simulink library "Mylibrary"  (Simulink 8.3)
settings: Solver=ode45  StartTime=0.0  StopTime=10.0  RelTol=1e-3
undefined symbols (not defined in the file or in its folder): Delay, epsilon, L, Mode, R, T_Trigger, tau_bar, Ts, Ts1, vd, Vehicle_Index, vp, x0, y0
undefined symbols (not defined in the file): d1, m1, psi20, Vx, Vy, x20, y20
libraries: Mylibrary x3
(part 1 of 3)
settings Model: Creator=hung  LastModifiedBy=hung  CovModelRefEnable=off  CovSFcnEnable=on

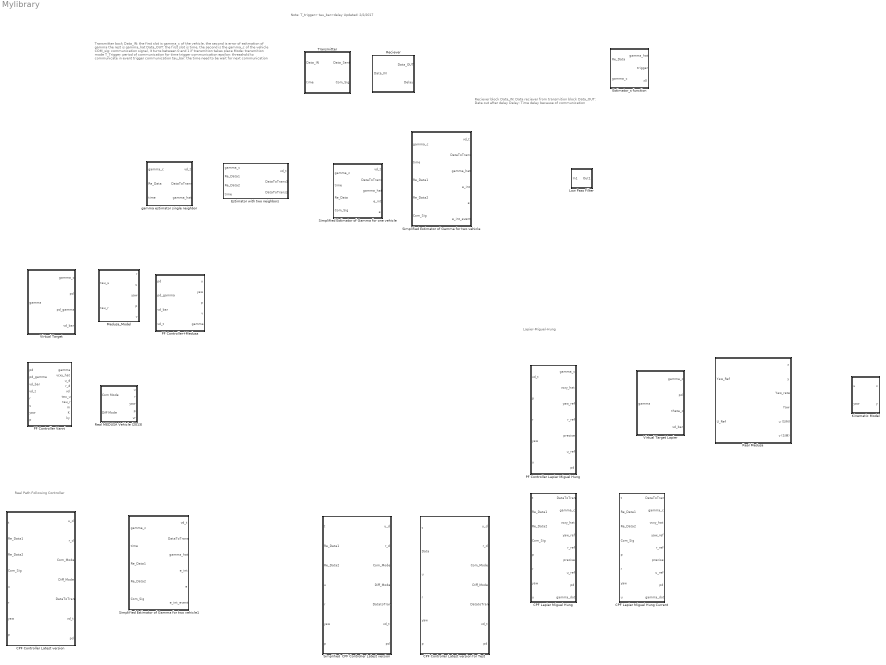
== system Mylibrary ==
  note: Lapier-Miguel-Hung
  note: Real Path Following Controller
  note: Note: T_trigger> tau_bar>delay
      | Updated: 2/2/2017
  note: Transmitter bock
      |
      | Data_IN: the first slot is gamma_c of the vehicle, the second is error of esitmation of gamma
      | the rest is gamma_hat
      | Data_OUT: the first slot is time, the second is the gamma_c of the vehicle
      | COM_sig: communication signal, it turns between 0 and 1 if transmition takes place
      |
      | Mode: transmition mode
      | T_Trigger: period of communication for time trigger communication
      | epsilon: threashold to communicate in event trigger communication
      | tau_bar: the time need to be wait for next communication
  note: Reciever block
      |
      | Data_IN: Data reciever from transmition block
      | Data_OUT: Data out after delay
      | Delay: Time delay because of communication
  " Real MEDUSA Vehicle (2013)" : Subsystem  mask{x0=0, y0=0, yaw0=0, u0=0, v0=0, r0=0, dist_u=0, dist_v=0, dist_r=0, Vcx=0, Vcy=0}
      mask prompts: dist_u "Disturbance in u"; dist_v "Disturbance in v"; dist_r "Disturbance in r"; Vcx "Current x"; Vcy "Current y"
  "CPF Controller Latest version  " : MATLAB Function  TreatAsAtomicUnit=on  mask{vp=0, L=0, m=0, d=0, R=0, tau_bar=0}
      settings: PermitHierarchicalResolution=ParametersOnly
  CPF Controller Latest version for Test : MATLAB Function  TreatAsAtomicUnit=on  mask{vp=0, L=0, m=0, d=0, R=0, tau_bar=0, Mode=0, T_Trigger=0, Parameter9=0, V_Id=0}
      mask prompts: Parameter9 "epsilon"
      settings: PermitHierarchicalResolution=ParametersOnly
  "CPF Lapier Miguel Hung " : MATLAB Function  TreatAsAtomicUnit=on  mask{L=L, R=R, d=d1, vp=vp, m=m1, tau_bar=tau_bar}
      settings: PermitHierarchicalResolution=ParametersOnly
  CPF Lapier Miguel Hung Current : MATLAB Function  TreatAsAtomicUnit=on  mask{L=L, R=R, d=d1, vp=vp, m=m1, tau_bar=tau_bar}
      settings: PermitHierarchicalResolution=ParametersOnly
  Estimator with two neighbors : Subsystem  mask{tau_bar=0, Parameter2=0}
      mask prompts: Parameter2 "Mode"
  Estimator_s function : Subsystem
  Kinematic Model : Subsystem
  Low Pass Filter : Subsystem
  Medusa_Model : Subsystem  mask{x0=x20, y0=y20, yaw0=psi20, u0=0, v0=0, r0=0, dist_u=0, dist_v=0, dist_r=0, Vcx=Vx, Vcy=Vy}
      mask prompts: dist_u "Disturbance in u"; dist_v "Disturbance in v"; dist_r "Disturbance in r"; Vcx "Current x"; Vcy "Current y"
  "PF Controller Lapier Miguel Hung " : MATLAB Function  TreatAsAtomicUnit=on  mask{L=L, R=R, d=d1, vd=vd, m=m1}
      settings: PermitHierarchicalResolution=ParametersOnly
  "PF Controller Vanni " : MATLAB Function  TreatAsAtomicUnit=on
      settings: PermitHierarchicalResolution=ParametersOnly
  PF Controller+Medusa : Subsystem
  Real Medusa : Subsystem
  Reciever : Subsystem  TreatAsAtomicUnit=on  mask{Delay=Delay}
      mask Display: image('Diagram2.png');
  "Simplified  CPF Controller Latest version " : MATLAB Function  TreatAsAtomicUnit=on  mask{vp=0, L=0, m=0, d=0, R=0, tau_bar=0, Mode=0, T_Trigger=0, Parameter9=0}
      mask prompts: Parameter9 "epsilon"
      settings: PermitHierarchicalResolution=ParametersOnly
  Simplified Estimator of Gamma for one vehicle : Subsystem  mask{Parameter1=0, Parameter2=0, Parameter3=0}
      mask prompts: Parameter1 "Mode"; Parameter2 "vd"; Parameter3 "tau_bar"
  Simplified Estimator of Gamma for two vehicle : Subsystem  mask{Parameter1=0, Parameter2=0, Parameter3=0}
      mask prompts: Parameter1 "Mode"; Parameter2 "vd"; Parameter3 "tau_bar"
  Simplified Estimator of Gamma for two vehicle1 : Subsystem  AncestorBlock=Mylibrary/Simplified Estimator of Gamma for two vehicle  mask{Parameter1=0, Parameter2=0, Parameter3=0}
      mask prompts: Parameter1 "Mode"; Parameter2 "vd"; Parameter3 "tau_bar"
  "Transmitter " : Subsystem  TreatAsAtomicUnit=on  mask{Mode=Mode, T_Trigger=T_Trigger, epsilon=epsilon, tau_bar=tau_bar}
      settings: MinAlgLoopOccurrences=on
      mask Display: image('transmit.png');
  Virtual Target : Subsystem  AncestorBlock=Mylibrary/Virtual Target  mask{L=0, R=0, d=0, vd=0, m=0}
      mask prompts: L "L (Length of the first segment)"; R "R (Radius for circumference)"; d "d (Offset from x axis)"; vd "vd (Speed profile)"
  Virtual Target Lapier : Subsystem  mask{L=0, R=0, d=0, vd=0, m=0}
      mask prompts: L "L (Length of the first segment)"; R "R (Radius for circumference)"; d "d (Offset from x axis)"; vd "vd (Speed profile)"
  gamma estimator single neighbor : Subsystem  TreatAsAtomicUnit=on  mask{Vehicle_Index=0, N_Vehicle_Index=0, tau_bar=0, Parameter4=0}
      mask prompts: Parameter4 "Mode"

== system Mylibrary/ Real MEDUSA Vehicle (2013) ==
  Com Mode : Inport
  Diff Mode : Inport  Port=2
  Medusa : Subsystem
  Mode : Constant  Value=4
  Mux : Mux  Inputs=2
  Saturation : Saturate  UpperLimit=100  LowerLimit=-100
  Saturation1 : Saturate  UpperLimit=100  LowerLimit=-100
  u : Outport
  r : Outport  Port=2
  yaw : Outport  Port=3
  p : Outport  Port=4
  vr : Outport  Port=5
  wires:
  Mode/1 -> Medusa/3(InnerLoops)
  Medusa/4(Yaw) -> yaw/1
  Medusa/3(Yaw_rate) -> r/1
  Medusa/6(v (SIM)) -> vr/1
  Medusa/5(u (SIM)) -> u/1
  Mux/1 -> p/1
  Medusa/1(x) -> Mux/1
  Medusa/2(y) -> Mux/2
  Diff Mode/1 -> Saturation1/1
  Com Mode/1 -> Saturation/1
  Saturation/1 -> Medusa/2(U_Ref)
  Saturation1/1 -> Medusa/1(Yaw_Ref)

== system Mylibrary/Estimator with two neighbors ==
  gamma_c : Inport
  Re_Data1 : Inport  Port=2
  Re_Data2 : Inport  Port=3
  time : Inport  Port=4
  Constant : Constant  Value=Mode
  Estimator i-j : Subsystem
  Estimator i-j1 : Mylibrary/Estimator with two neighbors/Estimator i-j
  MATLAB Function : MATLAB Function  TreatAsAtomicUnit=on
      settings: PermitHierarchicalResolution=ParametersOnly
  vd_t : Outport
  DataToTrans1 : Outport  Port=2
  DataToTrans2 : Outport  Port=3
  wires:
  time/1 -> Estimator i-j1/3, Estimator i-j/3("time ")
  gamma_c/1 -> Estimator i-j1/1, MATLAB Function/1(gamma_c), Estimator i-j/1(gamma_c)
  Estimator i-j1/2 -> MATLAB Function/3(gamma_hat2)
  Estimator i-j1/1 -> DataToTrans2/1
  Estimator i-j/1(DataToTrans) -> DataToTrans1/1
  Re_Data2/1 -> MATLAB Function/5(Re_Data2), Estimator i-j1/2
  Re_Data1/1 -> MATLAB Function/4(Re_Data1), Estimator i-j/2(Re_Data)
  Estimator i-j/2(gamma_hat) -> MATLAB Function/2(gamma_hat1)
  MATLAB Function/1(vd_t) -> vd_t/1
  Constant/1 -> MATLAB Function/6(Mode)

== system Mylibrary/Estimator_s function ==
  Re_Data : Inport
  gamma_c : Inport  Port=2
  Demux : Demux  Outputs=5
  Integrator : Integrator  ExternalReset=rising  InitialConditionSource=external
  Mux : Mux  Inputs=3
  Mux1 : Mux  Inputs=2
  Mux2 : Mux  Inputs=2
  S-Function : S-Function  FunctionName=estimator  Parameters=tau_bar  SFunctionDeploymentMode=off  EnableBusSupport=off
  gamma_hat : Outport
  trigger : Outport  Port=2
  x0 : Outport  Port=3
  wires:
  Mux1/1 -> x0/1, Integrator/3
  Mux/1 -> S-Function/1
  Demux/4 -> Mux1/1
  Demux/3 -> trigger/1, Integrator/2
  Mux2/1 -> Integrator/1
  S-Function/1 -> Demux/1
  Integrator/1 -> Mux/3, gamma_hat/1
  Demux/1 -> Mux2/1
  Demux/2 -> Mux2/2
  Demux/5 -> Mux1/2
  Re_Data/1 -> Mux/1
  gamma_c/1 -> Mux/2

== system Mylibrary/Kinematic Model ==
  u : Inport
  yaw : Inport  Port=2
  Integrator : Integrator  InitialCondition=x0
  Integrator1 : Integrator  InitialCondition=y0
  Kinematic Model : MATLAB Function  TreatAsAtomicUnit=on
      settings: PermitHierarchicalResolution=ParametersOnly
  x : Outport
  y : Outport  Port=2
  wires:
  yaw/1 -> Kinematic Model/2(yaw)
  u/1 -> Kinematic Model/1(u)
  Integrator1/1 -> y/1
  Kinematic Model/1(x_dot) -> Integrator/1
  Kinematic Model/2(y_dot) -> Integrator1/1
  Integrator/1 -> x/1

== system Mylibrary/Low Pass Filter ==
  In1 : Inport
  Demux : Demux  Outputs=2
  Mux : Mux  Inputs=2
  Transfer Fcn : TransferFcn  Denominator=[.2 1]
  Transfer Fcn1 : TransferFcn  Denominator=[.2 1]
  Out1 : Outport
  wires:
  Demux/2 -> Transfer Fcn1/1
  In1/1 -> Demux/1
  Demux/1 -> Transfer Fcn/1
  Transfer Fcn/1 -> Mux/1
  Mux/1 -> Out1/1
  Transfer Fcn1/1 -> Mux/2

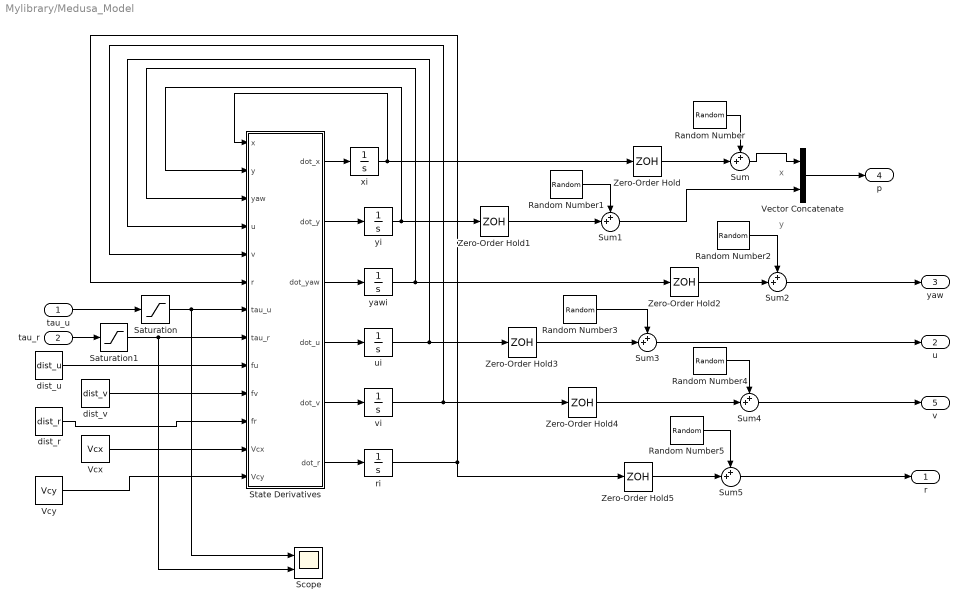
== system Mylibrary/Medusa_Model ==
  note: x
  note: y
  tau_u : Inport
  tau_r : Inport  Port=2
  Random Number : RandomNumber  Variance=.01  SampleTime=Ts1
  Random Number1 : RandomNumber  Variance=.01  SampleTime=Ts1
  Random Number2 : RandomNumber  Variance=.0001  SampleTime=Ts1
  Random Number3 : RandomNumber  Variance=.0001  SampleTime=Ts1
  Random Number4 : RandomNumber  SampleTime=Ts1
  Random Number5 : RandomNumber  Variance=0.0001  SampleTime=Ts1
  Saturation : Saturate  UpperLimit=100  LowerLimit=-100  ZeroCross=off
  Saturation1 : Saturate  UpperLimit=100  LowerLimit=-100  ZeroCross=off
  Scope : Scope  NumInputPorts=2
      settings: TimeRange=auto  MaxDataPoints=5000  SaveToWorkspace=off  SaveName=ScopeData3  YMin=-125.00000~-5  YMax=125.00000~5  SampleTime=-1
  State Derivatives : MATLAB Function  TreatAsAtomicUnit=on
      settings: PermitHierarchicalResolution=ParametersOnly
  Sum{,1..5} (6 alike) : Sum  Inputs=++|
  Vcx : Constant  Value=Vcx
  Vcy : Constant  Value=Vcy
  Vector Concatenate : Concatenate
  Zero-Order Hold{,1..5} (6 alike) : ZeroOrderHold  SampleTime=Ts1
  dist_r : Constant  Value=dist_r
  dist_u : Constant  Value=dist_u
  dist_v : Constant  Value=dist_v
  ri : Integrator  InitialCondition=r0
  ui : Integrator  InitialCondition=u0
  vi : Integrator  InitialCondition=v0
  xi : Integrator  InitialCondition=x0
  yawi : Integrator  InitialCondition=yaw0
  yi : Integrator  InitialCondition=y0
  r : Outport
  u : Outport  Port=2
  yaw : Outport  Port=3
  p : Outport  Port=4
  v : Outport  Port=5
  wires:
  State Derivatives/1(dot_x) -> xi/1
  State Derivatives/2(dot_y) -> yi/1
  State Derivatives/3(dot_yaw) -> yawi/1
  State Derivatives/4(dot_u) -> ui/1
  State Derivatives/5(dot_v) -> vi/1
  State Derivatives/6(dot_r) -> ri/1
  tau_u/1 -> Saturation/1
  tau_r/1 -> Saturation1/1
  dist_u/1 -> State Derivatives/9(fu)
  dist_v/1 -> State Derivatives/10(fv)
  dist_r/1 -> State Derivatives/11(fr)
  Vcx/1 -> State Derivatives/12(Vcx)
  Vcy/1 -> State Derivatives/13(Vcy)
  xi/1 -> Zero-Order Hold/1, State Derivatives/1(x)
  yi/1 -> Zero-Order Hold1/1, State Derivatives/2(y)
  ui/1 -> State Derivatives/4(u), Zero-Order Hold3/1
  vi/1 -> State Derivatives/5(v), Zero-Order Hold4/1
  ri/1 -> State Derivatives/6(r), Zero-Order Hold5/1
  Vector Concatenate/1 -> p/1
  Saturation/1 -> Scope/1, State Derivatives/7(tau_u)
  Saturation1/1 -> Scope/2, State Derivatives/8(tau_r)
  Sum1/1 -> Vector Concatenate/2
  Zero-Order Hold/1 -> Sum/2
  Sum/1 -> Vector Concatenate/1
  Random Number/1 -> Sum/1
  Zero-Order Hold1/1 -> Sum1/2
  Random Number1/1 -> Sum1/1
  yawi/1 -> Zero-Order Hold2/1, State Derivatives/3(yaw)
  Zero-Order Hold2/1 -> Sum2/2
  Sum2/1 -> yaw/1
  Random Number2/1 -> Sum2/1
  Zero-Order Hold3/1 -> Sum3/2
  Sum3/1 -> u/1
  Random Number3/1 -> Sum3/1
  Zero-Order Hold4/1 -> Sum4/2
  Sum4/1 -> v/1
  Random Number4/1 -> Sum4/1
  Zero-Order Hold5/1 -> Sum5/2
  Sum5/1 -> r/1
  Random Number5/1 -> Sum5/1

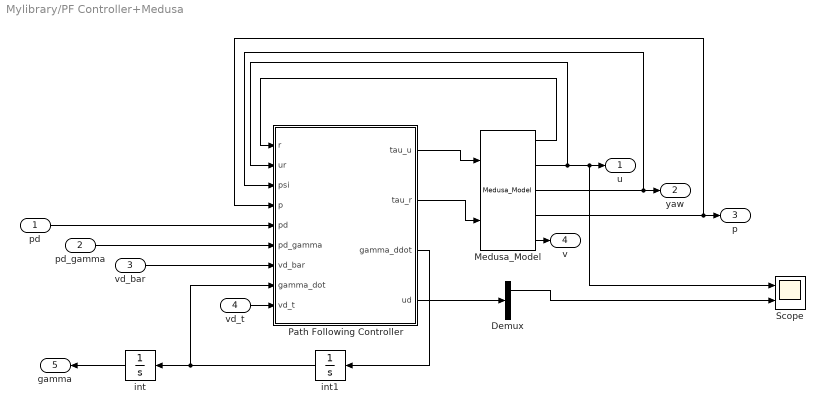
== system Mylibrary/PF Controller+Medusa ==
  pd : Inport
  pd_gamma : Inport  Port=2
  vd_bar : Inport  Port=3
  vd_t : Inport  Port=4
  Demux : Demux  Outputs=2
  Medusa_Model : Mylibrary/Medusa_Model  x0=x20  y0=y20  yaw0=psi20  u0=0  v0=0  r0=0  dist_u=0  dist_v=0  dist_r=0  Vcx=Vx  Vcy=Vy
  Path Following Controller : Subsystem
  Scope : Scope  NumInputPorts=2
      settings: TimeRange=auto  MaxDataPoints=5000  SaveToWorkspace=off  YMin=-1.16126~-5  YMax=10.45136~5  SampleTime=-1
  int : Integrator
  int1 : Integrator
  u : Outport
  yaw : Outport  Port=2
  p : Outport  Port=3
  v : Outport  Port=4
  gamma : Outport  Port=5
  wires:
  Medusa_Model/4 -> Path Following Controller/4(p), p/1
  Medusa_Model/3 -> Path Following Controller/3(psi), yaw/1
  Path Following Controller/3(gamma_ddot) -> int1/1
  pd/1 -> Path Following Controller/5(pd)
  int1/1 -> Path Following Controller/8(gamma_dot), int/1
  Path Following Controller/2(tau_r) -> Medusa_Model/2
  Medusa_Model/1 -> Path Following Controller/1(r)
  Medusa_Model/2 -> Path Following Controller/2(ur), Scope/1, u/1
  Path Following Controller/1(tau_u) -> Medusa_Model/1
  pd_gamma/1 -> Path Following Controller/6(pd_gamma)
  vd_bar/1 -> Path Following Controller/7(vd_bar)
  Medusa_Model/5 -> v/1
  vd_t/1 -> Path Following Controller/9(vd_t)
  int/1 -> gamma/1
  Path Following Controller/4(ud) -> Demux/1
  Demux/1 -> Scope/2

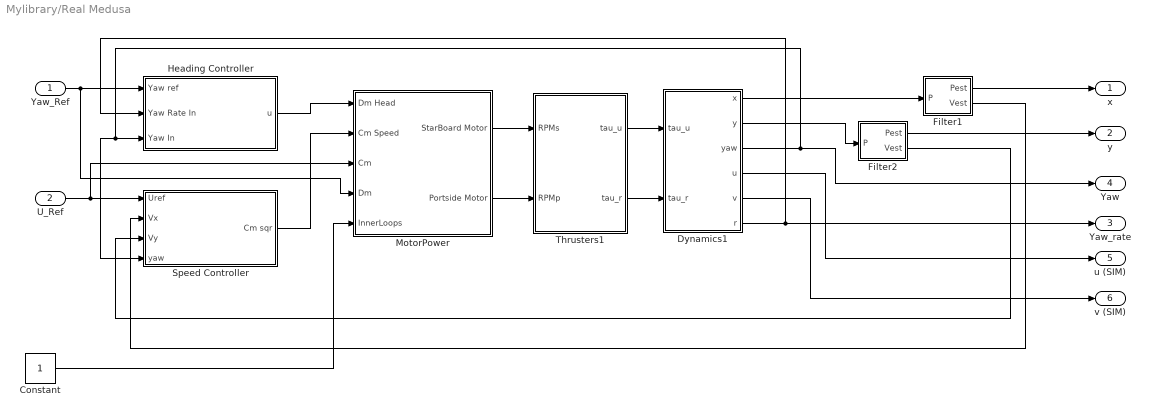
== system Mylibrary/Real Medusa ==
  Yaw_Ref : Inport
  U_Ref : Inport  Port=2
  Constant : Constant
  Dynamics1 : Subsystem  mask{x0=0, y0=0, yaw0=0, u0=0, v0=0, r0=0, dist_u=0, dist_v=0, dist_r=0, Vcx=0, Vcy=0}
      mask prompts: dist_u "Disturbance in u"; dist_v "Disturbance in v"; dist_r "Disturbance in r"; Vcx "Current x"; Vcy "Current y"
  Filter1 : Subsystem
  Filter2 : Subsystem
  Heading Controller : Subsystem  mask{Kp=45, Kd=110}
  MotorPower : Subsystem
  "Speed Controller " : Subsystem  mask{Kpu=60, Kiu=2, KSat=60}
      mask prompts: Kpu "Kp"; Kiu "Ki"; KSat "Common Mode Saturation"
  Thrusters1 : Subsystem
  x : Outport
  y : Outport  Port=2
  Yaw_rate : Outport  Port=3
  Yaw : Outport  Port=4
  u (SIM) : Outport  Port=5
  v (SIM) : Outport  Port=6
  wires:
  Thrusters1/1(tau_u) -> Dynamics1/1(tau_u)
  Thrusters1/2(tau_r) -> Dynamics1/2(tau_r)
  Dynamics1/1(x) -> Filter1/1(P)
  Dynamics1/2(y) -> Filter2/1(P)
  Dynamics1/3(yaw) -> Heading Controller/3(Yaw In), "Speed Controller "/4(yaw), Yaw/1
  MotorPower/1(StarBoard Motor) -> Thrusters1/1(RPMs)
  MotorPower/2(Portside Motor) -> Thrusters1/2(RPMp)
  Dynamics1/6(r) -> Heading Controller/2(Yaw Rate In), Yaw_rate/1
  Filter1/2(Vest) -> "Speed Controller "/2(Vx)
  Filter2/2(Vest) -> "Speed Controller "/3(Vy)
  "Speed Controller "/1(Cm sqr) -> MotorPower/2(Cm Speed)
  Yaw_Ref/1 -> Heading Controller/1(Yaw ref), MotorPower/4(Dm)
  Filter1/1(Pest) -> x/1
  Filter2/1(Pest) -> y/1
  U_Ref/1 -> "Speed Controller "/1(Uref), MotorPower/3(Cm)
  Heading Controller/1(u) -> MotorPower/1(Dm Head)
  Dynamics1/4(u) -> u (SIM)/1
  Dynamics1/5(v) -> v (SIM)/1
  Constant/1 -> MotorPower/5(InnerLoops)

== system Mylibrary/Reciever ==
  Data_IN : Inport  Priority=10
  Network Delay : MATLAB Function  Priority=11
      settings: PermitHierarchicalResolution=ParametersOnly
  Variable Time Delay1 : VariableTransportDelay  Priority=12  MaximumDelay=10  MaximumPoints=2048  ZeroDelay=on
  delay time : Constant  Value=Delay
  Data_OUT : Outport
  Delay : Outport  Port=2
  wires:
  Variable Time Delay1/1 -> Data_OUT/1
  delay time/1 -> Network Delay/2(DelayBound)
  Network Delay/1(delay_ins) -> Variable Time Delay1/2, Delay/1
  Data_IN/1 -> Variable Time Delay1/1, Network Delay/1(data)

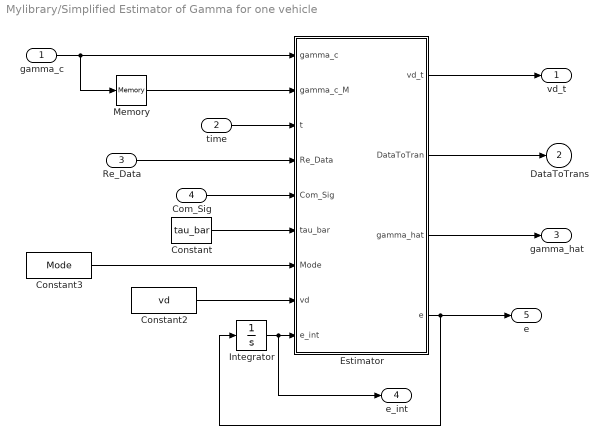
== system Mylibrary/Simplified Estimator of Gamma for one vehicle ==
  gamma_c : Inport
  "time " : Inport  Port=2
  Re_Data : Inport  Port=3
  Com_Sig : Inport  Port=4
  Constant : Constant  Value=tau_bar
  Constant2 : Constant  Value=vd
  Constant3 : Constant  Value=Mode
  Estimator : MATLAB Function  TreatAsAtomicUnit=on
      settings: PermitHierarchicalResolution=ParametersOnly
  Integrator : Integrator
  Memory : Memory
  vd_t : Outport
  DataToTrans : Outport  Port=2
  gamma_hat : Outport  Port=3
  e_int : Outport  Port=4
  e : Outport  Port=5
  wires:
  Constant3/1 -> Estimator/7(Mode)
  Estimator/2(DataToTran) -> DataToTrans/1
  Estimator/1(vd_t) -> vd_t/1
  Com_Sig/1 -> Estimator/5(Com_Sig)
  Re_Data/1 -> Estimator/4(Re_Data)
  "time "/1 -> Estimator/3(t)
  Constant/1 -> Estimator/6(tau_bar)
  Estimator/3(gamma_hat) -> gamma_hat/1
  Constant2/1 -> Estimator/8(vd)
  Estimator/4(e) -> e/1, Integrator/1
  Integrator/1 -> e_int/1, Estimator/9(e_int)
  gamma_c/1 -> Memory/1, Estimator/1(gamma_c)
  Memory/1 -> Estimator/2(gamma_c_M)

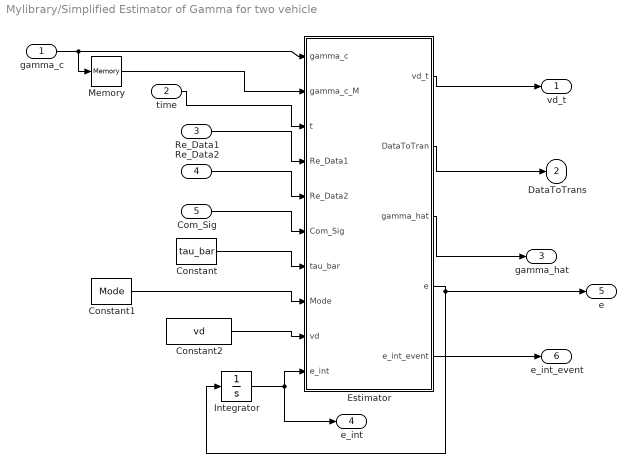
== system Mylibrary/Simplified Estimator of Gamma for two vehicle ==
  gamma_c : Inport
  "time " : Inport  Port=2
  Re_Data1 : Inport  Port=3
  Re_Data2 : Inport  Port=4
  Com_Sig : Inport  Port=5
  Constant : Constant  Value=tau_bar
  Constant1 : Constant  Value=Mode
  Constant2 : Constant  Value=vd
  Estimator : MATLAB Function  TreatAsAtomicUnit=on
      settings: PermitHierarchicalResolution=ParametersOnly
  Integrator : Integrator
  Memory : Memory
  vd_t : Outport
  DataToTrans : Outport  Port=2
  gamma_hat : Outport  Port=3
  e_int : Outport  Port=4
  e : Outport  Port=5
  e_int_event : Outport  Port=6
  wires:
  Estimator/1(vd_t) -> vd_t/1
  Estimator/3(gamma_hat) -> gamma_hat/1
  Constant2/1 -> Estimator/9(vd)
  Re_Data1/1 -> Estimator/4(Re_Data1)
  "time "/1 -> Estimator/3(t)
  Constant/1 -> Estimator/7(tau_bar)
  Com_Sig/1 -> Estimator/6(Com_Sig)
  Estimator/2(DataToTran) -> DataToTrans/1
  Re_Data2/1 -> Estimator/5(Re_Data2)
  Estimator/4(e) -> e/1, Integrator/1
  Integrator/1 -> e_int/1, Estimator/10(e_int)
  gamma_c/1 -> Memory/1, Estimator/1(gamma_c)
  Constant1/1 -> Estimator/8(Mode)
  Memory/1 -> Estimator/2(gamma_c_M)
  Estimator/5(e_int_event) -> e_int_event/1

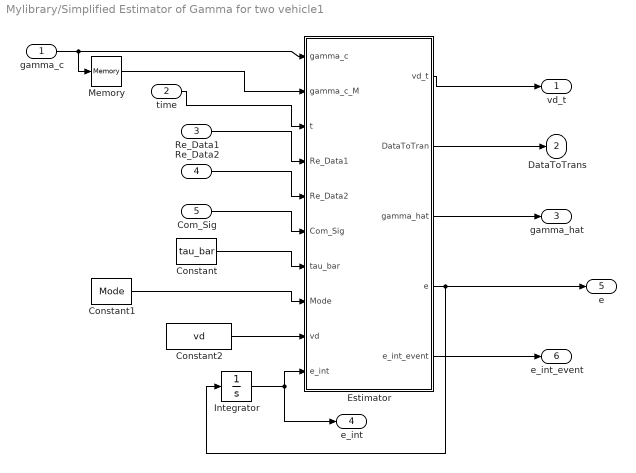
== system Mylibrary/Simplified Estimator of Gamma for two vehicle1 ==
  gamma_c : Inport
  "time " : Inport  Port=2
  Re_Data1 : Inport  Port=3
  Re_Data2 : Inport  Port=4
  Com_Sig : Inport  Port=5
  Constant : Constant  Value=tau_bar
  Constant1 : Constant  Value=Mode
  Constant2 : Constant  Value=vd
  Estimator : MATLAB Function  TreatAsAtomicUnit=on
      settings: PermitHierarchicalResolution=ParametersOnly
  Integrator : Integrator
  Memory : Memory
  vd_t : Outport
  DataToTrans : Outport  Port=2
  gamma_hat : Outport  Port=3
  e_int : Outport  Port=4
  e : Outport  Port=5
  e_int_event : Outport  Port=6
  wires:
  Estimator/1(vd_t) -> vd_t/1
  Estimator/3(gamma_hat) -> gamma_hat/1
  Constant2/1 -> Estimator/9(vd)
  Re_Data1/1 -> Estimator/4(Re_Data1)
  "time "/1 -> Estimator/3(t)
  Constant/1 -> Estimator/7(tau_bar)
  Com_Sig/1 -> Estimator/6(Com_Sig)
  Estimator/2(DataToTran) -> DataToTrans/1
  Re_Data2/1 -> Estimator/5(Re_Data2)
  Estimator/4(e) -> Integrator/1, e/1
  Integrator/1 -> e_int/1, Estimator/10(e_int)
  gamma_c/1 -> Memory/1, Estimator/1(gamma_c)
  Constant1/1 -> Estimator/8(Mode)
  Memory/1 -> Estimator/2(gamma_c_M)
  Estimator/5(e_int_event) -> e_int_event/1

== system Mylibrary/Transmitter  ==
  Data_IN : Inport
  time : Inport  Port=2
  Constant : Constant  Value=Mode
  Constant1 : Constant  Value=T_Trigger
  Constant2 : Constant  Value=epsilon
  Constant3 : Constant  Value=tau_bar
  Transmitter : MATLAB Function  TreatAsAtomicUnit=on
      settings: PermitHierarchicalResolution=ParametersOnly  MinAlgLoopOccurrences=on
  Unit Delay : UnitDelay  SampleTime=0.2
  Unit Delay1 : UnitDelay  SampleTime=0.2
  Data_Sent : Outport
  Com_Sig : Outport  Port=2
  wires:
  Data_IN/1 -> Transmitter/2(Data_IN)
  time/1 -> Transmitter/1(t)
  Constant/1 -> Transmitter/3(Mode)
  Constant1/1 -> Transmitter/4(T_Trigger)
  Constant2/1 -> Transmitter/5(epsilon)
  Constant3/1 -> Transmitter/6(tau_bar)
  Transmitter/1(Data_OUT) -> Unit Delay/1
  Transmitter/2(Comm_Sig) -> Unit Delay1/1
  Unit Delay/1 -> Data_Sent/1
  Unit Delay1/1 -> Com_Sig/1

== system Mylibrary/Virtual Target ==
  gamma : Inport
  L : Constant  Value=L
  R : Constant  Value=R
  Virtual Target Position 2 : MATLAB Function  TreatAsAtomicUnit=on
      settings: PermitHierarchicalResolution=ParametersOnly
  d : Constant  Value=d
  m : Constant  Value=m
  vd : Constant  Value=vd
  gamma_c : Outport
  pd : Outport  Port=2
  pd_gamma : Outport  Port=3
  vd_bar : Outport  Port=4
  wires:
  R/1 -> Virtual Target Position 2/4(R)
  Virtual Target Position 2/3(pd_gamma) -> pd_gamma/1
  Virtual Target Position 2/4(vd_bar) -> vd_bar/1
  Virtual Target Position 2/1(gamma_c) -> gamma_c/1
  Virtual Target Position 2/2(pd) -> pd/1
  gamma/1 -> Virtual Target Position 2/1(gamma)
  L/1 -> Virtual Target Position 2/3(L)
  vd/1 -> Virtual Target Position 2/2(vd)
  d/1 -> Virtual Target Position 2/5(d)
  m/1 -> Virtual Target Position 2/6(m)

== system Mylibrary/Virtual Target Lapier ==
  gamma : Inport
  L : Constant  Value=L
  R : Constant  Value=R
  Virtual Target Position 2 : MATLAB Function  TreatAsAtomicUnit=on
      settings: PermitHierarchicalResolution=ParametersOnly
  d : Constant  Value=d
  m : Constant  Value=m
  vd : Constant  Value=vd
  gamma_c : Outport
  pd : Outport  Port=2
  theta_c : Outport  Port=3
  vd_bar : Outport  Port=4
  wires:
  R/1 -> Virtual Target Position 2/4(R)
  Virtual Target Position 2/4(theta_c) -> theta_c/1
  Virtual Target Position 2/3(vd_bar) -> vd_bar/1
  Virtual Target Position 2/1(gamma_c) -> gamma_c/1
  Virtual Target Position 2/2(pd) -> pd/1
  gamma/1 -> Virtual Target Position 2/1(gamma)
  L/1 -> Virtual Target Position 2/3(L)
  vd/1 -> Virtual Target Position 2/2(vd)
  d/1 -> Virtual Target Position 2/5(d)
  m/1 -> Virtual Target Position 2/6(m)

== system Mylibrary/gamma estimator single neighbor ==
  gamma_c : Inport
  Re_Data : Inport  Port=2
  "time " : Inport  Port=3
  Constant : Constant  Value=tau_bar
  Constant1 : Constant  Value=Vehicle_Index
  Constant3 : Constant  Value=Mode
  Estimator : MATLAB Function  TreatAsAtomicUnit=on
      settings: PermitHierarchicalResolution=ParametersOnly
  Integrator : Integrator  ExternalReset=rising  InitialConditionSource=external
  vd_t : Outport
  DataToTrans : Outport  Port=2
  gamma_hat : Outport  Port=3
  wires:
  Estimator/2(trigger) -> Integrator/2
  Estimator/3(x0) -> Integrator/3
  gamma_c/1 -> Estimator/3(gamma_c)
  Estimator/1(gamma_dot) -> Integrator/1
  Integrator/1 -> gamma_hat/1, Estimator/6(gamma_hat)
  Constant/1 -> Estimator/4(tau_bar)
  "time "/1 -> Estimator/1(t)
  Re_Data/1 -> Estimator/2(Re_Data)
  Constant1/1 -> Estimator/5(Vehicle_Index)
  Estimator/4(vd_t) -> vd_t/1
  Estimator/5(DataToTran) -> DataToTrans/1
  Constant3/1 -> Estimator/7(Mode)

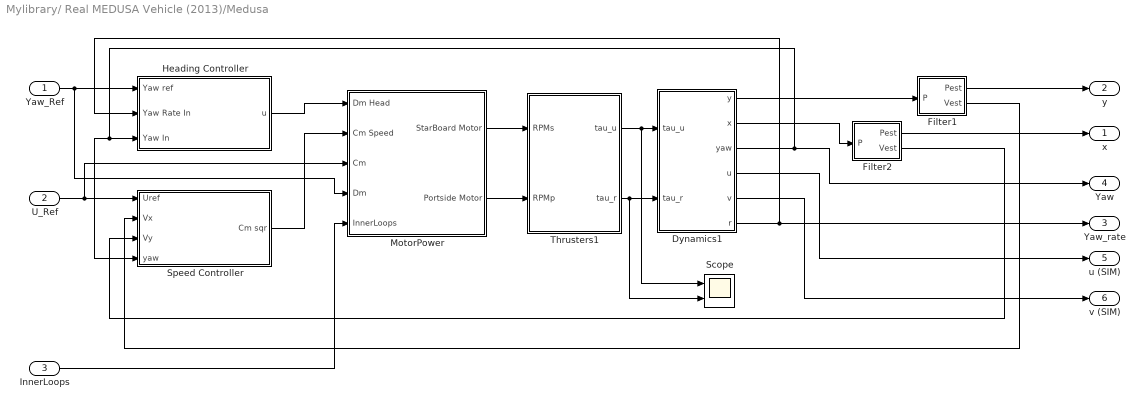
== system Mylibrary/ Real MEDUSA Vehicle (2013)/Medusa ==
  Yaw_Ref : Inport
  U_Ref : Inport  Port=2
  InnerLoops : Inport  Port=3
  Dynamics1 : Subsystem
  Filter1 : Subsystem
  Filter2 : Subsystem
  Heading Controller : Subsystem  mask{Kp=45, Kd=110}
  MotorPower : Subsystem
  Scope : Scope  NumInputPorts=2
      settings: TimeRange=auto  MaxDataPoints=5000  SaveToWorkspace=off  YMin=-10~-5  YMax=10~5  SampleTime=-1
  "Speed Controller " : Subsystem  mask{Kpu=60, Kiu=2, KSat=60}
      mask prompts: Kpu "Kp"; Kiu "Ki"; KSat "Common Mode Saturation"
  Thrusters1 : Subsystem
  x : Outport
  y : Outport  Port=2
  Yaw_rate : Outport  Port=3
  Yaw : Outport  Port=4
  u (SIM) : Outport  Port=5
  v (SIM) : Outport  Port=6
  wires:
  Thrusters1/1(tau_u) -> Scope/1, Dynamics1/1(tau_u)
  Thrusters1/2(tau_r) -> Scope/2, Dynamics1/2(tau_r)
  Dynamics1/1(y) -> Filter1/1(P)
  Dynamics1/2(x) -> Filter2/1(P)
  Dynamics1/3(yaw) -> Heading Controller/3(Yaw In), "Speed Controller "/4(yaw), Yaw/1
  MotorPower/1(StarBoard Motor) -> Thrusters1/1(RPMs)
  MotorPower/2(Portside Motor) -> Thrusters1/2(RPMp)
  Dynamics1/6(r) -> Heading Controller/2(Yaw Rate In), Yaw_rate/1
  Filter1/2(Vest) -> "Speed Controller "/2(Vx)
  Filter2/2(Vest) -> "Speed Controller "/3(Vy)
  "Speed Controller "/1(Cm sqr) -> MotorPower/2(Cm Speed)
  Yaw_Ref/1 -> Heading Controller/1(Yaw ref), MotorPower/4(Dm)
  Filter1/1(Pest) -> y/1
  Filter2/1(Pest) -> x/1
  U_Ref/1 -> "Speed Controller "/1(Uref), MotorPower/3(Cm)
  Heading Controller/1(u) -> MotorPower/1(Dm Head)
  InnerLoops/1 -> MotorPower/5(InnerLoops)
  Dynamics1/4(u) -> u (SIM)/1
  Dynamics1/5(v) -> v (SIM)/1

== system Mylibrary/Estimator with two neighbors/Estimator i-j ==
  gamma_c : Inport
  Re_Data : Inport  Port=2
  "time " : Inport  Port=3
  Constant : Constant  Value=tau_bar
  Constant1 : Constant  Value=Vehicle_Index
  Estimator : MATLAB Function  TreatAsAtomicUnit=on
      settings: PermitHierarchicalResolution=ParametersOnly
  Integrator : Integrator  ExternalReset=rising  InitialConditionSource=external
  DataToTrans : Outport
  gamma_hat : Outport  Port=2
  wires:
  Re_Data/1 -> Estimator/2(Re_Data)
  "time "/1 -> Estimator/1(t)
  Estimator/4(DataToTran) -> DataToTrans/1
  Integrator/1 -> gamma_hat/1, Estimator/6(gamma_hat)
  Constant/1 -> Estimator/4(tau_bar)
  Estimator/1(gamma_dot) -> Integrator/1
  Constant1/1 -> Estimator/5(Vehicle_Index)
  gamma_c/1 -> Estimator/3(gamma_c)
  Estimator/3(x0) -> Integrator/3
  Estimator/2(trigger) -> Integrator/2

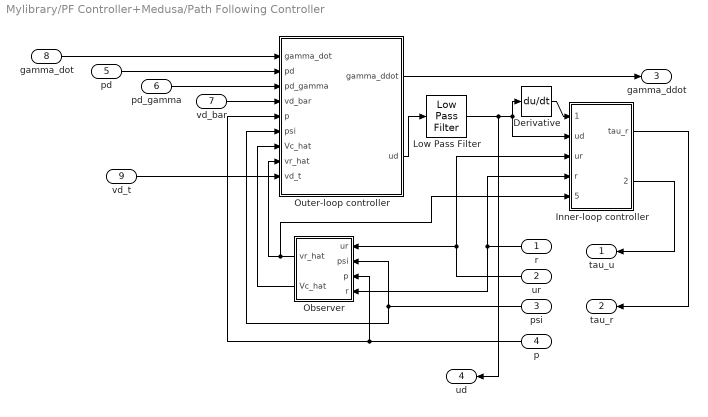
== system Mylibrary/PF Controller+Medusa/Path Following Controller ==
  r : Inport
  ur : Inport  Port=2
  psi : Inport  Port=3
  p : Inport  Port=4
  pd : Inport  Port=5
  pd_gamma : Inport  Port=6
  vd_bar : Inport  Port=7
  gamma_dot : Inport  Port=8
  vd_t : Inport  Port=9
  Derivative : Derivative
  Inner-loop controller : MATLAB Function  TreatAsAtomicUnit=on
      settings: PermitHierarchicalResolution=ParametersOnly
  Low Pass Filter : Mylibrary/Low Pass Filter
  Observer : Subsystem
  Outer-loop controller : MATLAB Function  TreatAsAtomicUnit=on
      settings: PermitHierarchicalResolution=ParametersOnly
  tau_u : Outport
  tau_r : Outport  Port=2
  gamma_ddot : Outport  Port=3
  ud : Outport  Port=4
  wires:
  Inner-loop controller/2(tau_u) -> tau_u/1
  Inner-loop controller/1(tau_r) -> tau_r/1
  r/1 -> Observer/4(r), Inner-loop controller/4(r)
  ur/1 -> Observer/1(ur), Inner-loop controller/3(ur)
  Outer-loop controller/2(ud) -> Low Pass Filter/1
  Observer/2(Vc_hat) -> Outer-loop controller/7(Vc_hat)
  psi/1 -> Outer-loop controller/6(psi), Observer/2(psi)
  p/1 -> Observer/3(p), Outer-loop controller/5(p)
  pd/1 -> Outer-loop controller/2(pd)
  pd_gamma/1 -> Outer-loop controller/3(pd_gamma)
  vd_bar/1 -> Outer-loop controller/4(vd_bar)
  Observer/1(vr_hat) -> Inner-loop controller/5(vr_hat), Outer-loop controller/8(vr_hat)
  Outer-loop controller/1(gamma_ddot) -> gamma_ddot/1
  gamma_dot/1 -> Outer-loop controller/1(gamma_dot)
  Derivative/1 -> Inner-loop controller/1(ud_dot)
  vd_t/1 -> Outer-loop controller/9(vd_t)
  Low Pass Filter/1 -> ud/1, Inner-loop controller/2(ud), Derivative/1

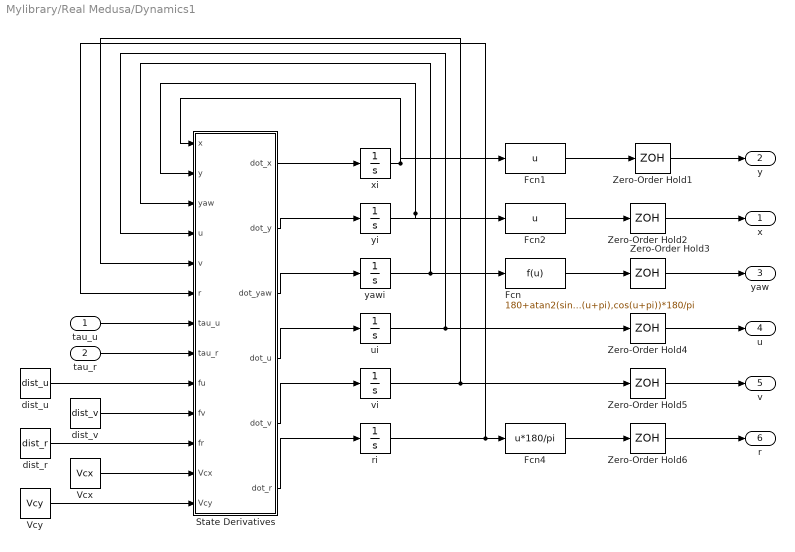
== system Mylibrary/Real Medusa/Dynamics1 ==
  tau_u : Inport
  tau_r : Inport  Port=2
  Fcn : Fcn  Expr=180+atan2(sin(u+pi),cos(u+pi))*180/pi
  Fcn1 : Fcn  Expr=u
  Fcn2 : Fcn  Expr=u
  Fcn4 : Fcn  Expr=u*180/pi
  State Derivatives : MATLAB Function  TreatAsAtomicUnit=on
      settings: PermitHierarchicalResolution=ParametersOnly
  Vcx : Constant  Value=Vcx
  Vcy : Constant  Value=Vcy
  Zero-Order Hold{1..6} (6 alike) : ZeroOrderHold  SampleTime=0.2
  dist_r : Constant  Value=dist_r
  dist_u : Constant  Value=dist_u
  dist_v : Constant  Value=dist_v
  ri : Integrator  InitialCondition=r0
  ui : Integrator  InitialCondition=u0
  vi : Integrator  InitialCondition=v0
  xi : Integrator  InitialCondition=y0
  yawi : Integrator  InitialCondition=yaw0
  yi : Integrator  InitialCondition=x0
  x : Outport
  y : Outport  Port=2
  yaw : Outport  Port=3
  u : Outport  Port=4
  v : Outport  Port=5
  r : Outport  Port=6
  wires:
  Fcn4/1 -> Zero-Order Hold6/1
  State Derivatives/1(dot_x) -> xi/1
  State Derivatives/2(dot_y) -> yi/1
  State Derivatives/3(dot_yaw) -> yawi/1
  State Derivatives/4(dot_u) -> ui/1
  State Derivatives/5(dot_v) -> vi/1
  State Derivatives/6(dot_r) -> ri/1
  tau_u/1 -> State Derivatives/7(tau_u)
  yi/1 -> State Derivatives/2(y), Fcn2/1
  xi/1 -> State Derivatives/1(x), Fcn1/1
  yawi/1 -> Fcn/1, State Derivatives/3(yaw)
  ui/1 -> State Derivatives/4(u), Zero-Order Hold4/1
  ri/1 -> Fcn4/1, State Derivatives/6(r)
  vi/1 -> State Derivatives/5(v), Zero-Order Hold5/1
  tau_r/1 -> State Derivatives/8(tau_r)
  dist_u/1 -> State Derivatives/9(fu)
  dist_v/1 -> State Derivatives/10(fv)
  dist_r/1 -> State Derivatives/11(fr)
  Fcn/1 -> Zero-Order Hold3/1
  Vcx/1 -> State Derivatives/12(Vcx)
  Vcy/1 -> State Derivatives/13(Vcy)
  Fcn1/1 -> Zero-Order Hold1/1
  Fcn2/1 -> Zero-Order Hold2/1
  Zero-Order Hold1/1 -> y/1
  Zero-Order Hold2/1 -> x/1
  Zero-Order Hold3/1 -> yaw/1
  Zero-Order Hold4/1 -> u/1
  Zero-Order Hold5/1 -> v/1
  Zero-Order Hold6/1 -> r/1

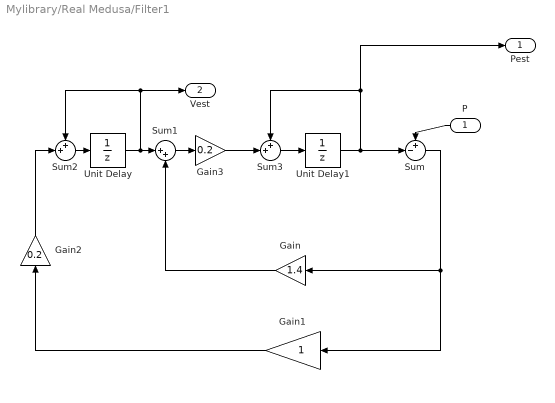
== system Mylibrary/Real Medusa/Filter1 ==
  P : Inport
  Gain : Gain  Gain=1.4
  Gain1 : Gain
  Gain2 : Gain  Gain=0.2
  Gain3 : Gain  Gain=0.2
  Sum : Sum  Inputs=+-|
  Sum1 : Sum  Inputs=|++
  Sum2 : Sum  Inputs=++|
  Sum3 : Sum  Inputs=++|
  Unit Delay : UnitDelay  SampleTime=-1
  Unit Delay1 : UnitDelay  SampleTime=-1
  Pest : Outport
  Vest : Outport  Port=2
  wires:
  Sum3/1 -> Unit Delay1/1
  Unit Delay1/1 -> Pest/1, Sum3/1, Sum/2
  Gain3/1 -> Sum3/2
  Gain2/1 -> Sum2/2
  Sum2/1 -> Unit Delay/1
  P/1 -> Sum/1
  Gain1/1 -> Gain2/1
  Unit Delay/1 -> Vest/1, Sum2/1, Sum1/1
  Gain/1 -> Sum1/2
  Sum/1 -> Gain1/1, Gain/1
  Sum1/1 -> Gain3/1

== system Mylibrary/Real Medusa/Filter2 ==
  P : Inport
  Gain : Gain  Gain=1.4
  Gain1 : Gain
  Gain2 : Gain  Gain=0.2
  Gain3 : Gain  Gain=0.2
  Sum : Sum  Inputs=+-|
  Sum1 : Sum  Inputs=|++
  Sum2 : Sum  Inputs=++|
  Sum3 : Sum  Inputs=++|
  Unit Delay : UnitDelay  SampleTime=-1
  Unit Delay1 : UnitDelay  SampleTime=-1
  Pest : Outport
  Vest : Outport  Port=2
  wires:
  Sum1/1 -> Gain3/1
  Sum/1 -> Gain/1, Gain1/1
  Gain/1 -> Sum1/2
  Unit Delay/1 -> Sum1/1, Sum2/1, Vest/1
  Gain1/1 -> Gain2/1
  P/1 -> Sum/1
  Sum2/1 -> Unit Delay/1
  Gain2/1 -> Sum2/2
  Gain3/1 -> Sum3/2
  Unit Delay1/1 -> Sum/2, Sum3/1, Pest/1
  Sum3/1 -> Unit Delay1/1

== system Mylibrary/Real Medusa/Heading Controller ==
  note: 0-360
  note: Saida em Percentagem
  Yaw ref : Inport  SampleTime=Ts
  Yaw Rate In : Inport  Port=2  SampleTime=Ts
  Yaw In : Inport  Port=3
  Embedded MATLAB Function1 : MATLAB Function  TreatAsAtomicUnit=on
      settings: PermitHierarchicalResolution=ParametersOnly
  sat : Saturate  UpperLimit=Inf  LowerLimit=-Inf  SampleTime=Ts
  u : Outport
  wires:
  Yaw ref/1 -> Embedded MATLAB Function1/1(YawRef)
  Embedded MATLAB Function1/1(x) -> sat/1
  Yaw In/1 -> Embedded MATLAB Function1/2(Yaw)
  Yaw Rate In/1 -> Embedded MATLAB Function1/3(Yawrate)
  sat/1 -> u/1

== system Mylibrary/Real Medusa/MotorPower ==
  Dm Head : Inport
  Cm Speed : Inport  Port=2
  Cm : Inport  Port=3
  Dm : Inport  Port=4
  InnerLoops : Inport  Port=5
  Embedded MATLAB Function : MATLAB Function  TreatAsAtomicUnit=on
      settings: PermitHierarchicalResolution=ParametersOnly
  StarBoard Motor : Outport
  Portside Motor : Outport  Port=2
  wires:
  Embedded MATLAB Function/2(Pm) -> Portside Motor/1
  Embedded MATLAB Function/1(Sm) -> StarBoard Motor/1
  Dm Head/1 -> Embedded MATLAB Function/2(Dm_Head)
  Cm Speed/1 -> Embedded MATLAB Function/1(Cm_Speed)
  Cm/1 -> Embedded MATLAB Function/3(Cm)
  Dm/1 -> Embedded MATLAB Function/4(Dm)
  InnerLoops/1 -> Embedded MATLAB Function/5(InnerLoops)

== system Mylibrary/Real Medusa/Speed Controller  ==
  Uref : Inport
  Vx : Inport  Port=2
  Vy : Inport  Port=3
  yaw : Inport  Port=4
  Embedded MATLAB Function1 : MATLAB Function  TreatAsAtomicUnit=on
      settings: PermitHierarchicalResolution=ParametersOnly
  Scope4 : Scope
      settings: TimeRange=auto  LimitDataPoints=on  MaxDataPoints=5000  SaveToWorkspace=off  SaveName=ScopeData5  YMin=-10  YMax=10  SampleTime=-1
  Smith Predictor : Subsystem
  Unit Delay : UnitDelay  SampleTime=0.2
  sqr : Fcn  Expr=abs(u)*u
  Cm sqr : Outport
  wires:
  Embedded MATLAB Function1/3(u) -> Scope4/1
  yaw/1 -> Embedded MATLAB Function1/5(yaw)
  Vy/1 -> Embedded MATLAB Function1/4(Vy)
  Vx/1 -> Embedded MATLAB Function1/3(Vx)
  Embedded MATLAB Function1/1(Cm) -> Smith Predictor/1(Cm), sqr/1
  Uref/1 -> Embedded MATLAB Function1/1(Uref)
  Embedded MATLAB Function1/2(qsi) -> Unit Delay/1
  Unit Delay/1 -> Embedded MATLAB Function1/2(qsiold)
  sqr/1 -> Cm sqr/1

== system Mylibrary/Real Medusa/Thrusters1 ==
  RPMs : Inport
  RPMp : Inport  Port=2
  Add : Sum
  Add1 : Sum  Inputs=-+
  Motor Port : Subsystem  mask{K0=7.2115, tau=0.346, eta=4/(1500^2)}
      mask prompts: tau "Atraso do Motor"; eta "Constante de conversao W-F"
  Motor Stardboard : Subsystem  mask{K0=7.2115, tau=0.346, eta=4/(1500^2)}
      mask prompts: tau "Atraso do Motor"; eta "Constante de conversao W-F"
  l : Gain  Gain=0.25
  tau_u : Outport
  tau_r : Outport  Port=2
  wires:
  Add1/1 -> l/1
  RPMs/1 -> Motor Stardboard/1(w RPM)
  Add/1 -> tau_u/1
  RPMp/1 -> Motor Port/1(w RPM)
  l/1 -> tau_r/1
  Motor Port/1(F) -> Add/2, Add1/2
  Motor Stardboard/1(F) -> Add/1, Add1/1

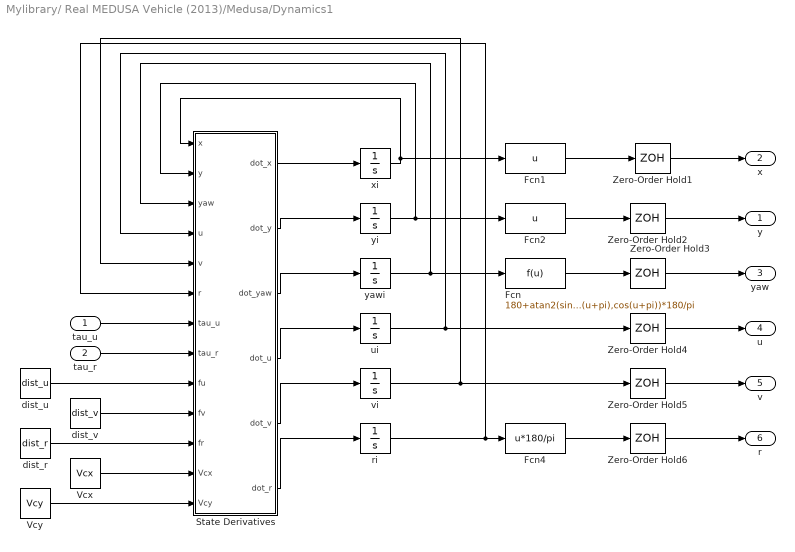
== system Mylibrary/ Real MEDUSA Vehicle (2013)/Medusa/Dynamics1 ==
  tau_u : Inport
  tau_r : Inport  Port=2
  Fcn : Fcn  Expr=180+atan2(sin(u+pi),cos(u+pi))*180/pi
  Fcn1 : Fcn  Expr=u
  Fcn2 : Fcn  Expr=u
  Fcn4 : Fcn  Expr=u*180/pi
  State Derivatives : MATLAB Function  TreatAsAtomicUnit=on
      settings: PermitHierarchicalResolution=ParametersOnly
  Vcx : Constant  Value=Vcx
  Vcy : Constant  Value=Vcy
  Zero-Order Hold{1..6} (6 alike) : ZeroOrderHold  SampleTime=0.2
  dist_r : Constant  Value=dist_r
  dist_u : Constant  Value=dist_u
  dist_v : Constant  Value=dist_v
  ri : Integrator  InitialCondition=r0
  ui : Integrator  InitialCondition=u0
  vi : Integrator  InitialCondition=v0
  xi : Integrator  InitialCondition=x0
  yawi : Integrator  InitialCondition=yaw0
  yi : Integrator  InitialCondition=y0
  y : Outport
  x : Outport  Port=2
  yaw : Outport  Port=3
  u : Outport  Port=4
  v : Outport  Port=5
  r : Outport  Port=6
  wires:
  Fcn4/1 -> Zero-Order Hold6/1
  State Derivatives/1(dot_x) -> xi/1
  State Derivatives/2(dot_y) -> yi/1
  State Derivatives/3(dot_yaw) -> yawi/1
  State Derivatives/4(dot_u) -> ui/1
  State Derivatives/5(dot_v) -> vi/1
  State Derivatives/6(dot_r) -> ri/1
  tau_u/1 -> State Derivatives/7(tau_u)
  yi/1 -> State Derivatives/2(y), Fcn2/1
  xi/1 -> State Derivatives/1(x), Fcn1/1
  yawi/1 -> Fcn/1, State Derivatives/3(yaw)
  ui/1 -> State Derivatives/4(u), Zero-Order Hold4/1
  ri/1 -> Fcn4/1, State Derivatives/6(r)
  vi/1 -> State Derivatives/5(v), Zero-Order Hold5/1
  tau_r/1 -> State Derivatives/8(tau_r)
  dist_u/1 -> State Derivatives/9(fu)
  dist_v/1 -> State Derivatives/10(fv)
  dist_r/1 -> State Derivatives/11(fr)
  Fcn/1 -> Zero-Order Hold3/1
  Vcx/1 -> State Derivatives/12(Vcx)
  Vcy/1 -> State Derivatives/13(Vcy)
  Fcn1/1 -> Zero-Order Hold1/1
  Fcn2/1 -> Zero-Order Hold2/1
  Zero-Order Hold1/1 -> x/1
  Zero-Order Hold2/1 -> y/1
  Zero-Order Hold3/1 -> yaw/1
  Zero-Order Hold4/1 -> u/1
  Zero-Order Hold5/1 -> v/1
  Zero-Order Hold6/1 -> r/1

== system Mylibrary/ Real MEDUSA Vehicle (2013)/Medusa/Filter1 ==
  P : Inport
  Gain : Gain  Gain=1.4
  Gain1 : Gain
  Gain2 : Gain  Gain=0.2
  Gain3 : Gain  Gain=0.2
  Sum : Sum  Inputs=+-|
  Sum1 : Sum  Inputs=|++
  Sum2 : Sum  Inputs=++|
  Sum3 : Sum  Inputs=++|
  Unit Delay : UnitDelay  SampleTime=-1
  Unit Delay1 : UnitDelay  SampleTime=-1
  Pest : Outport
  Vest : Outport  Port=2
  wires:
  Sum3/1 -> Unit Delay1/1
  Unit Delay1/1 -> Pest/1, Sum3/1, Sum/2
  Gain3/1 -> Sum3/2
  Gain2/1 -> Sum2/2
  Sum2/1 -> Unit Delay/1
  P/1 -> Sum/1
  Gain1/1 -> Gain2/1
  Unit Delay/1 -> Vest/1, Sum2/1, Sum1/1
  Gain/1 -> Sum1/2
  Sum/1 -> Gain1/1, Gain/1
  Sum1/1 -> Gain3/1

== system Mylibrary/ Real MEDUSA Vehicle (2013)/Medusa/Filter2 ==
  P : Inport
  Gain : Gain  Gain=1.4
  Gain1 : Gain
  Gain2 : Gain  Gain=0.2
  Gain3 : Gain  Gain=0.2
  Sum : Sum  Inputs=+-|
  Sum1 : Sum  Inputs=|++
  Sum2 : Sum  Inputs=++|
  Sum3 : Sum  Inputs=++|
  Unit Delay : UnitDelay  SampleTime=-1
  Unit Delay1 : UnitDelay  SampleTime=-1
  Pest : Outport
  Vest : Outport  Port=2
  wires:
  Sum1/1 -> Gain3/1
  Sum/1 -> Gain/1, Gain1/1
  Gain/1 -> Sum1/2
  Unit Delay/1 -> Sum1/1, Sum2/1, Vest/1
  Gain1/1 -> Gain2/1
  P/1 -> Sum/1
  Sum2/1 -> Unit Delay/1
  Gain2/1 -> Sum2/2
  Gain3/1 -> Sum3/2
  Unit Delay1/1 -> Sum/2, Sum3/1, Pest/1
  Sum3/1 -> Unit Delay1/1

== system Mylibrary/ Real MEDUSA Vehicle (2013)/Medusa/Heading Controller ==
  note: 0-360
  note: Saida em Percentagem
  Yaw ref : Inport  SampleTime=Ts
  Yaw Rate In : Inport  Port=2  SampleTime=Ts
  Yaw In : Inport  Port=3
  Embedded MATLAB Function1 : MATLAB Function  TreatAsAtomicUnit=on
      settings: PermitHierarchicalResolution=ParametersOnly
  sat : Saturate  UpperLimit=Inf  LowerLimit=-Inf  SampleTime=Ts
  u : Outport
  wires:
  Yaw ref/1 -> Embedded MATLAB Function1/1(YawRef)
  Embedded MATLAB Function1/1(x) -> sat/1
  Yaw In/1 -> Embedded MATLAB Function1/2(Yaw)
  Yaw Rate In/1 -> Embedded MATLAB Function1/3(Yawrate)
  sat/1 -> u/1

== system Mylibrary/ Real MEDUSA Vehicle (2013)/Medusa/MotorPower ==
  Dm Head : Inport
  Cm Speed : Inport  Port=2
  Cm : Inport  Port=3
  Dm : Inport  Port=4
  InnerLoops : Inport  Port=5
  Embedded MATLAB Function : MATLAB Function  TreatAsAtomicUnit=on
      settings: PermitHierarchicalResolution=ParametersOnly
  StarBoard Motor : Outport
  Portside Motor : Outport  Port=2
  wires:
  Embedded MATLAB Function/2(Pm) -> Portside Motor/1
  Embedded MATLAB Function/1(Sm) -> StarBoard Motor/1
  Dm Head/1 -> Embedded MATLAB Function/2(Dm_Head)
  Cm Speed/1 -> Embedded MATLAB Function/1(Cm_Speed)
  Cm/1 -> Embedded MATLAB Function/3(Cm)
  Dm/1 -> Embedded MATLAB Function/4(Dm)
  InnerLoops/1 -> Embedded MATLAB Function/5(InnerLoops)

== system Mylibrary/ Real MEDUSA Vehicle (2013)/Medusa/Speed Controller  ==
  Uref : Inport
  Vx : Inport  Port=2
  Vy : Inport  Port=3
  yaw : Inport  Port=4
  Embedded MATLAB Function1 : MATLAB Function  TreatAsAtomicUnit=on
      settings: PermitHierarchicalResolution=ParametersOnly
  Scope4 : Scope
      settings: TimeRange=auto  LimitDataPoints=on  MaxDataPoints=5000  SaveToWorkspace=off  SaveName=ScopeData5  YMin=-10  YMax=10  SampleTime=-1
  Smith Predictor : Subsystem
  Unit Delay : UnitDelay  SampleTime=0.2
  sqr : Fcn  Expr=abs(u)*u
  Cm sqr : Outport
  wires:
  Embedded MATLAB Function1/3(u) -> Scope4/1
  yaw/1 -> Embedded MATLAB Function1/5(yaw)
  Vy/1 -> Embedded MATLAB Function1/4(Vy)
  Vx/1 -> Embedded MATLAB Function1/3(Vx)
  Embedded MATLAB Function1/1(Cm) -> Smith Predictor/1(Cm), sqr/1
  Uref/1 -> Embedded MATLAB Function1/1(Uref)
  Embedded MATLAB Function1/2(qsi) -> Unit Delay/1
  Unit Delay/1 -> Embedded MATLAB Function1/2(qsiold)
  sqr/1 -> Cm sqr/1

== system Mylibrary/ Real MEDUSA Vehicle (2013)/Medusa/Thrusters1 ==
  RPMs : Inport
  RPMp : Inport  Port=2
  Add : Sum
  Add1 : Sum  Inputs=-+
  Motor Port : Subsystem  mask{K0=7.2115, tau=0.346, eta=4/(1500^2)}
      mask prompts: tau "Atraso do Motor"; eta "Constante de conversao W-F"
  Motor Stardboard : Subsystem  mask{K0=7.2115, tau=0.346, eta=4/(1500^2)}
      mask prompts: tau "Atraso do Motor"; eta "Constante de conversao W-F"
  l : Gain  Gain=0.25
  tau_u : Outport
  tau_r : Outport  Port=2
  wires:
  Add1/1 -> l/1
  RPMs/1 -> Motor Stardboard/1(w RPM)
  Add/1 -> tau_u/1
  RPMp/1 -> Motor Port/1(w RPM)
  l/1 -> tau_r/1
  Motor Port/1(F) -> Add/2, Add1/2
  Motor Stardboard/1(F) -> Add/1, Add1/1

== system Mylibrary/PF Controller+Medusa/Path Following Controller/Observer ==
  ur : Inport
  psi : Inport  Port=2
  p : Inport  Port=3  PortDimensions=2
  r : Inport  Port=4
  Unit Delay : UnitDelay  SampleTime=-1
  Unit Delay1 : UnitDelay  SampleTime=-1
  Unit Delay2 : UnitDelay  SampleTime=-1
  "observer of current and vr " : MATLAB Function  TreatAsAtomicUnit=on
      settings: PermitHierarchicalResolution=ParametersOnly
  vr_hat : Outport
  Vc_hat : Outport  Port=2
  wires:
  p/1 -> "observer of current and vr "/4(p)
  psi/1 -> "observer of current and vr "/3(psi)
  ur/1 -> "observer of current and vr "/2(ur)
  Unit Delay/1 -> "observer of current and vr "/6(p_hat_old)
  "observer of current and vr "/3(Vcxy_hat) -> Unit Delay1/1
  "observer of current and vr "/2(Vc_hat) -> Vc_hat/1
  "observer of current and vr "/4(p_hat) -> Unit Delay/1
  Unit Delay1/1 -> "observer of current and vr "/5(Vcxy_hat_old)
  "observer of current and vr "/1(vr_hat) -> vr_hat/1, Unit Delay2/1
  Unit Delay2/1 -> "observer of current and vr "/1(vr_hat_old)
  r/1 -> "observer of current and vr "/7(r)

== system Mylibrary/Real Medusa/Speed Controller /Smith Predictor ==
  Cm : Inport
  Common mode to u : DiscreteTransferFcn  Numerator=[0.0006641 0]  Denominator=[1 -0.6368 -0.2936]  SampleTime=0.2
  Integer Delay2 : Delay  DelayLength=7  InputProcessing=Inherited  SampleTime=0.2
  Sum2 : Sum  Inputs=|-+
  u : Outport
  wires:
  Cm/1 -> Common mode to u/1
  Common mode to u/1 -> Integer Delay2/1, Sum2/2
  Integer Delay2/1 -> Sum2/1
  Sum2/1 -> u/1

== system Mylibrary/Real Medusa/Thrusters1/Motor Port ==
  note: 100% -> 4500 rpm
  w RPM : Inport
  "  " : Rounding  Operator=round
  "  1" : Rounding  Operator=round
  Gain : Gain  Gain=45
  Sat [-100,100] : Saturate  UpperLimit=100  LowerLimit=-100
  "Sat [-100,100] " : Saturate  UpperLimit=100  LowerLimit=-100
  Transfer Fcn : TransferFcn  Numerator=[K0]  Denominator=[1 K0]
  Transport Delay : TransportDelay  DelayTime=tau
  "rpm -> N" : Fcn  Expr=eta * abs(u)* u
  F : Outport
  wires:
  Transfer Fcn/1 -> "  "/1
  Transport Delay/1 -> Transfer Fcn/1
  "  1"/1 -> Transport Delay/1
  "  "/1 -> "Sat [-100,100] "/1
  "rpm -> N"/1 -> F/1
  Sat [-100,100]/1 -> "  1"/1
  Gain/1 -> "rpm -> N"/1
  w RPM/1 -> Sat [-100,100]/1
  "Sat [-100,100] "/1 -> Gain/1

== system Mylibrary/Real Medusa/Thrusters1/Motor Stardboard ==
  note: 100% -> 4500 rpm
  w RPM : Inport
  "  " : Rounding  Operator=round
  "  1" : Rounding  Operator=round
  Aproximation : Fcn  Expr=eta * abs(u)* u
  Gain : Gain  Gain=45
  Saturation : Saturate  UpperLimit=100  LowerLimit=-100
  Saturation1 : Saturate  UpperLimit=100  LowerLimit=-100
  Transfer Fcn : TransferFcn  Numerator=[K0]  Denominator=[1 K0]
  Transport Delay : TransportDelay  DelayTime=tau
  F : Outport
  wires:
  Transfer Fcn/1 -> "  "/1
  Transport Delay/1 -> Transfer Fcn/1
  "  1"/1 -> Transport Delay/1
  "  "/1 -> Saturation/1
  Aproximation/1 -> F/1
  Saturation1/1 -> "  1"/1
  Gain/1 -> Aproximation/1
  w RPM/1 -> Saturation1/1
  Saturation/1 -> Gain/1

== system Mylibrary/ Real MEDUSA Vehicle (2013)/Medusa/Speed Controller /Smith Predictor ==
  Cm : Inport
  Common mode to u : DiscreteTransferFcn  Numerator=[0.0006641 0]  Denominator=[1 -0.6368 -0.2936]  SampleTime=0.2
  Integer Delay2 : Delay  DelayLength=7  InputProcessing=Inherited  SampleTime=0.2
  Sum2 : Sum  Inputs=|-+
  u : Outport
  wires:
  Cm/1 -> Common mode to u/1
  Common mode to u/1 -> Integer Delay2/1, Sum2/2
  Integer Delay2/1 -> Sum2/1
  Sum2/1 -> u/1

== system Mylibrary/ Real MEDUSA Vehicle (2013)/Medusa/Thrusters1/Motor Port ==
  note: 100% -> 4500 rpm
  w RPM : Inport
  "  " : Rounding  Operator=round
  "  1" : Rounding  Operator=round
  Gain : Gain  Gain=45
  Sat [-100,100] : Saturate  UpperLimit=100  LowerLimit=-100
  "Sat [-100,100] " : Saturate  UpperLimit=100  LowerLimit=-100
  Transfer Fcn : TransferFcn  Numerator=[K0]  Denominator=[1 K0]
  Transport Delay : TransportDelay  DelayTime=tau
  "rpm -> N" : Fcn  Expr=eta * abs(u)* u
  F : Outport
  wires:
  Transfer Fcn/1 -> "  "/1
  Transport Delay/1 -> Transfer Fcn/1
  "  1"/1 -> Transport Delay/1
  "  "/1 -> "Sat [-100,100] "/1
  "rpm -> N"/1 -> F/1
  Sat [-100,100]/1 -> "  1"/1
  Gain/1 -> "rpm -> N"/1
  w RPM/1 -> Sat [-100,100]/1
  "Sat [-100,100] "/1 -> Gain/1

== system Mylibrary/ Real MEDUSA Vehicle (2013)/Medusa/Thrusters1/Motor Stardboard ==
  note: 100% -> 4500 rpm
  w RPM : Inport
  "  " : Rounding  Operator=round
  "  1" : Rounding  Operator=round
  Aproximation : Fcn  Expr=eta * abs(u)* u
  Gain : Gain  Gain=45
  Saturation : Saturate  UpperLimit=100  LowerLimit=-100
  Saturation1 : Saturate  UpperLimit=100  LowerLimit=-100
  Transfer Fcn : TransferFcn  Numerator=[K0]  Denominator=[1 K0]
  Transport Delay : TransportDelay  DelayTime=tau
  F : Outport
  wires:
  Transfer Fcn/1 -> "  "/1
  Transport Delay/1 -> Transfer Fcn/1
  "  1"/1 -> Transport Delay/1
  "  "/1 -> Saturation/1
  Aproximation/1 -> F/1
  Saturation1/1 -> "  1"/1
  Gain/1 -> Aproximation/1
  w RPM/1 -> Saturation1/1
  Saturation/1 -> Gain/1

== matlab function Reciever/Network Delay ==
  settings: updateMethod=DISCRETE  sampleTime=.01
  data: data input double size=2; delay_ins output double; DelayBound input double; Mode input double
function delay_ins = fcn(data,DelayBound,Mode)
persistent delay;
persistent data_old;
if isempty(delay)
    delay=0;
    data_old=0;
end
if (data(1)~=0)
    delay=DelayBound*round(10*rand)/10;
%     delay=0.6;
end
data_old=data(2);
if Mode==0
    delay=0;
end
delay_ins=delay;                                 % Instance delay;

== matlab function Estimator with two neighbors/Estimator i-j/Estimator ==
  data: t input double; Re_Data input double; gamma_dot output double; gamma_c input double; trigger output double; x0 output double; tau_bar input double; Vehicle_Index input double; gamma_hat input double size=2; DataToTran output double size=4
function [gamma_dot,trigger,x0,DataToTran] = fcn(t,Re_Data,gamma_c,tau_bar,Vehicle_Index,gamma_hat)

%% compute error term of velocity 
% kg=0.3;
vd=1;kg=0.05;
L=[1 -1;
   -1 1]; 
% trigger=Re_Data(2); 
% x0=[gamma_c;Re_Data(2)];
% gamma_dot = vd*[1;1];

%% Reset estimator of gamma
persistent data_old t_recieve trigger_tem gamma_n;   
if isempty(data_old)
    data_old=Re_Data(1);
    t_recieve=t;
    trigger_tem=0;
    gamma_n=0;
end
if (Re_Data(1)~=0)
    t_recieve=Re_Data(1);
    trigger_tem=0;
    gamma_n=Re_Data(2)+vd*tau_bar;
end   
if (t-t_recieve>tau_bar)
    trigger_tem=1;
end
data_old=Re_Data(1);


x0=[gamma_c;gamma_n];
trigger=trigger_tem;
% gamma_dot = vd*[1;1]-kg*L*gamma_hat;
gamma_dot = vd*[1;1];

% %% Compute correction term 
% if Mode==0;
%     gamma_c_n_hat=Re_Data(2);
% else
%     gamma_c_n_hat=gamma_hat(2);
% end
% % gamma_c_hat=gamma_hat(Vehicle_Index);
% vd_t=-kg*(gamma_c-gamma_c_n_hat);  
%% Prepare Data for transmition block
gamma_e=gamma_c-gamma_hat(1);
DataToTran=[gamma_c;gamma_e;gamma_hat];

== matlab function Transmitter /Transmitter ==
  settings: updateMethod=DISCRETE  sampleTime=0.01
  data: t input double; Data_IN input double size=2; Mode input double; T_Trigger input double; epsilon input double; tau_bar input double; Data_OUT output double size=2; Comm_Sig output double
function [Data_OUT,Comm_Sig]  = fcn(t,Data_IN,Mode,T_Trigger,epsilon,tau_bar)
%% Initialize temporary variables
persistent t_sent;
emptydata=[0;0]; 
gamma_c=Data_IN(1);            
gamma_e=Data_IN(2);
if isempty(t_sent);
    t_sent=-tau_bar;
    Data_OUT=emptydata;
    Comm_Sig=0;
else
    Data_OUT=emptydata;
    Comm_Sig=1;
end

% Time trigger communication
if Mode==1                                  
   if ~mod(t,T_Trigger)                           
        Data_OUT=[t;gamma_c];     
        t_sent=t;  % Include time in transmitted data
        Comm_Sig=1;
   else
        Data_OUT=emptydata;
        Comm_Sig=0;
   end           
end
 t_wait=t-t_sent;
if Mode==2                                  
    if ((abs(gamma_e)>=epsilon)&&(t_wait>=0.2));      % Event trigger 
        t_sent=t;                                 % Taged t to t_sent;     
        Data_OUT=[t;gamma_c];
        Comm_Sig=1;
    else 
        Data_OUT=emptydata;
        Comm_Sig=0;
    end
end

== matlab function Estimator with two neighbors/MATLAB Function ==
  data: gamma_c input double; vd_t output double; gamma_hat1 input double; gamma_hat2 input double; Re_Data1 input double; Re_Data2 input double; Mode input double
function vd_t = fcn(gamma_c,gamma_hat1,gamma_hat2,Re_Data1,Re_Data2,Mode)
%#codegen
kg=0.05;
if Mode==0
    vd_t=-kg*(gamma_c-0.5*(Re_Data1(2)+Re_Data2(2)));
else
    vd_t=-kg*(gamma_c-0.5*(gamma_hat1(2)+gamma_hat2(2)));
end

== matlab function Simplified Estimator of Gamma for one vehicle/Estimator ==
  data: vd_t output double size=1; DataToTran output double size=2; gamma_c input double; gamma_c_M input double; t input double; Re_Data input double size=2; Com_Sig input double; gamma_hat output double; tau_bar input double; Mode input double; vd input double; e_int input double; e output double
function [vd_t,DataToTran,gamma_hat,e] = fcn(gamma_c,gamma_c_M,t,Re_Data,Com_Sig,tau_bar,Mode,vd,e_int)

%% 
kg=1;
% L=[1 -1;
%    -1 1]; 

%% Reset estimator of gamma
persistent gamma_cn0 gamma_c0 tc1 tc2 tcn1 tcn2 tem_c tem_cn reset_c reset_cn;   
if isempty(gamma_cn0)
    gamma_cn0=0;
    gamma_c0=0;
    tcn1=t;
    tcn2=t;
    tc1=t;
    tc2=t;
    tem_c=0;
    tem_cn=0;
    reset_c=false;
    reset_cn=false;
end
%% Reset estimator for gamma_c of neighbor;
if (Re_Data(1)~=0)                                  % If recived new data, reset estimator that the current vehicle thinks about the neighbor vehicle
    tcn1=Re_Data(1); 
    tem_cn=Re_Data(2);
    reset_cn=true;
end   
if (t-tcn1>tau_bar)&&reset_cn                        % Reset gamma after waiting time tau_bar
    gamma_cn0=tem_cn+vd*tau_bar;
    reset_cn=false;
    tcn2=t;
end
%% Reset estimator for gamma_c of current vehicle  
if (Com_Sig~=0)                                     % When it sends its coordinate state to neighbor, it needs to update its estimator too to synchoronize with the neighbor
    tc1=t;
    tem_c=gamma_c;
    reset_c=true;
end
if (t-tc1>tau_bar)&& reset_c                        % Reset gamma after waiting for time tau_bar 
    gamma_c0=tem_c+vd*tau_bar;
    reset_c=false;
    tc2=t;
end
%% Run estimators
gamma_c_hat=gamma_c0+vd*(t-tc2);
gamma_c_n_hat=gamma_cn0+vd*(t-tcn2);
gamma_hat=[gamma_c_hat;gamma_c_n_hat]; 
ki=10;
if Mode==0
    e=gamma_c_M-Re_Data(2);
else
   if (Re_Data(1)~=0)  
        e=gamma_c_M-Re_Data(2);
   else
        e=0;
   end
end

%% Compute correction term 
if Mode==0;          % if Mode==0, continous communication, we use direct data recieved from neighbor.
    vd_t=-kg*e-ki*e_int; 
else
    vd_t=-kg*(gamma_c-gamma_c_n_hat)-ki*e_int;
end
 
%% Prepare Data for transmition block
gamma_e=gamma_c-gamma_c_hat;
% DataToTran=[gamma_c;gamma_e;gamma_hat];
DataToTran=[gamma_c;gamma_e];
